simulink model "model"  (R2023b)
settings: Solver=VariableStepAuto  StartTime=0.0  StopTime=10.0  RelTol=1e-3
settings Model: Creator=student  LastModifiedBy=student

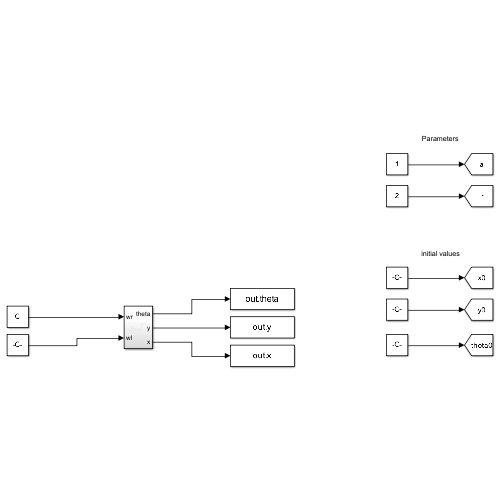
[thumbnail: Simulink's stored preview of the top-level diagram]
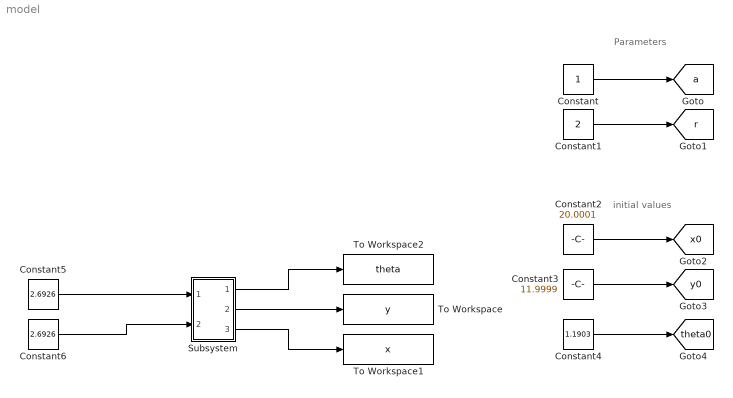
== system model ==
  note: initial values
  note: Parameters
  Constant : Constant
  Constant1 : Constant  Value=2
  Constant2 : Constant  Value=20.0001
  Constant3 : Constant  Value=11.9999
  Constant4 : Constant  Value=1.1903
  Constant5 : Constant  Value=2.6926
  Constant6 : Constant  Value=2.6926
  Subsystem : Subsystem
  To Workspace : ToWorkspace  VariableName=y  SampleTime=-1
  To Workspace1 : ToWorkspace  VariableName=x  SampleTime=-1
  To Workspace2 : ToWorkspace  VariableName=theta  SampleTime=-1
  tag scope: a=global, r=global, theta0=global, x0=global, y0=global
  wires:
  Constant/1 -> [a]
  Constant1/1 -> [r]
  Constant2/1 -> [x0]
  Constant3/1 -> [y0]
  Constant4/1 -> [theta0]
  Constant5/1 -> Subsystem/1(In1)
  Constant6/1 -> Subsystem/2(In2)
  Subsystem/2(Out2) -> To Workspace/1
  Subsystem/3(Out3) -> To Workspace1/1
  Subsystem/1(Out1) -> To Workspace2/1

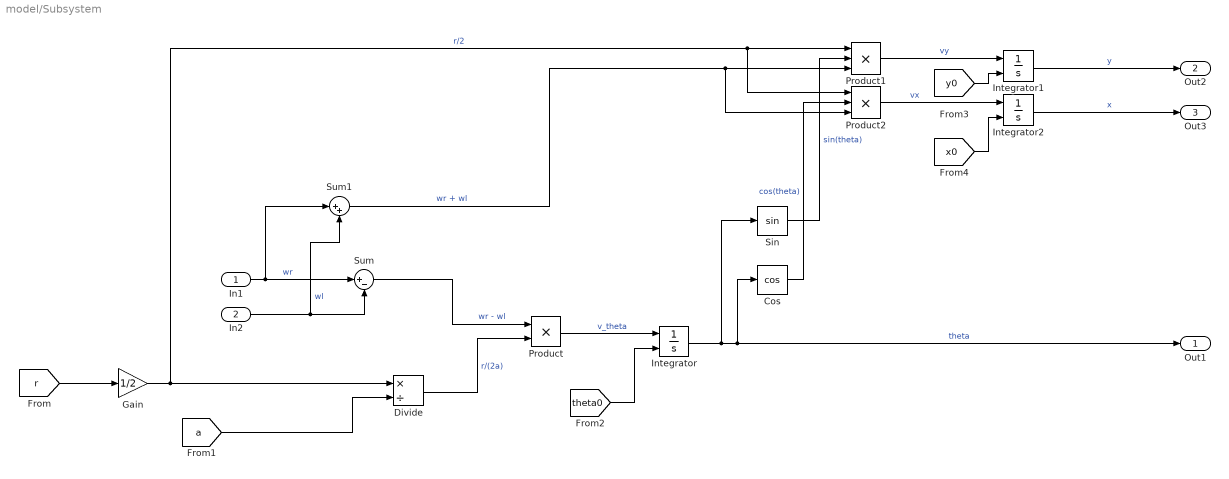
== system model/Subsystem ==
  In1 : Inport
  In2 : Inport  Port=2
  Cos : Trigonometry  Operator=cos
  Divide : Product  Inputs=*/
  Gain : Gain  Gain=1/2
  Integrator : Integrator  InitialConditionSource=external
  Integrator1 : Integrator  InitialConditionSource=external
  Integrator2 : Integrator  InitialConditionSource=external
  Product : Product
  Product1 : Product  Inputs=3
  Product2 : Product  Inputs=3
  Sin : Trigonometry
  Sum : Sum  Inputs=|+-
  Sum1 : Sum  Inputs=|++
  Out1 : Outport
  Out2 : Outport  Port=2
  Out3 : Outport  Port=3
  wires:
  In1/1 -> Sum1/1, Sum/1  "wr"
  In2/1 -> Sum1/2, Sum/2  "wl"
  Gain/1 -> Product2/1, Product1/1, Divide/1  "r/2"
  [r] -> Gain/1
  [a] -> Divide/2
  Divide/1 -> Product/2  "r/(2a)"
  Sum/1 -> Product/1  "wr - wl"
  Sum1/1 -> Product2/3, Product1/3  "wr + wl"
  Product/1 -> Integrator/1  "v_theta"
  Integrator/1 -> Sin/1, Cos/1, Out1/1  "theta"
  [theta0] -> Integrator/2
  Cos/1 -> Product2/2  "cos(theta)"
  Sin/1 -> Product1/2  "sin(theta)"
  Product2/1 -> Integrator2/1  "vx"
  Product1/1 -> Integrator1/1  "vy"
  [x0] -> Integrator2/2
  [y0] -> Integrator1/2
  Integrator1/1 -> Out2/1  "y"
  Integrator2/1 -> Out3/1  "x"
